simulink model "Ball_Estimation_10_12"  (Simulink 8.1)
settings: Solver=ode4  StartTime=0.0  StopTime=inf  FixedStep=sample_time  RelTol=1e-3
InitFcn:
  | sample_time=0.005;%0.004;%0.0025;%0.02;
  | sample_time_Vicon = 0.005;
  | DeltaT = 0.02;
  | g = 9.81;
  | H0 = g%0.3165;
  | Kl = 1;
  | 
  | Omega_r = 1.6;%for Horizontal reference
  | Zeta_r = 0.7; %for Horizontal reference
  | Omega = 1.8;%for Horizontal Control
  | Zeta = 0.5;    %for Horizontal Control
  | 
  | Omega_h_r = 2.2; %for vertical reference
  | Zeta_h_r = 0.8;  %for vertical reference
  | Omega_h = 2.3;    %for vertical control
  | Zeta_h = 0.8;         %for vertical control
  | PI=pi;
  | 
  | Mass = 1;
  | Acc_Max = 4;
  | Acc_Max_h = 4;
  | 
  | Max_RP = 60;
  | 
  | % for NN
  | n = 5;
  | r = 3;
  | n2 = 5;
  | NN_ST = 0.02;
  | 
  | GAMA_V = 6;
  | gama_V_e = 0.01;
  | 
  | GAMA_W = GAMA_V;
  | gama_W_e =0.01;
  | 
  | % deadzone
  | NN_Deadzone_Z = 0;
  | 
  | % inputs nomalizaton parameters
  | NN_Z_y_min = -3;
  | NN_Z_y_max = 0.5;
  | 
  | NN_Z_v_max = 8;
  | NN_Z_v_min = -NN_Z_v_max;
  | 
  | % alpha = 0.034;
  | alpha = 1;
  | % c_f = 0.0015;
  | c_f = 0.001;
  | c_y_tilt = 1*0.5;
undefined symbols (not defined in the file or in its folder): DiscIntNeverNeededParam
undefined symbols (not defined in the file): Q6_acc_max, Q6_acc_max_h, Q6_Omega_r, Q6_Omega_r_h, Q6_Zeta_r, Q6_Zeta_r_h
libraries: X330_Control x4, simulink x4
settings Model: Creator=ttcl3  LastModifiedBy=Vicon
settings SolverCC: MaxConsecutiveMinStep=auto
settings DebuggingCC: MultiTaskRateTransMsg=warning
settings SFSimCC: SimParseCustomCode=off

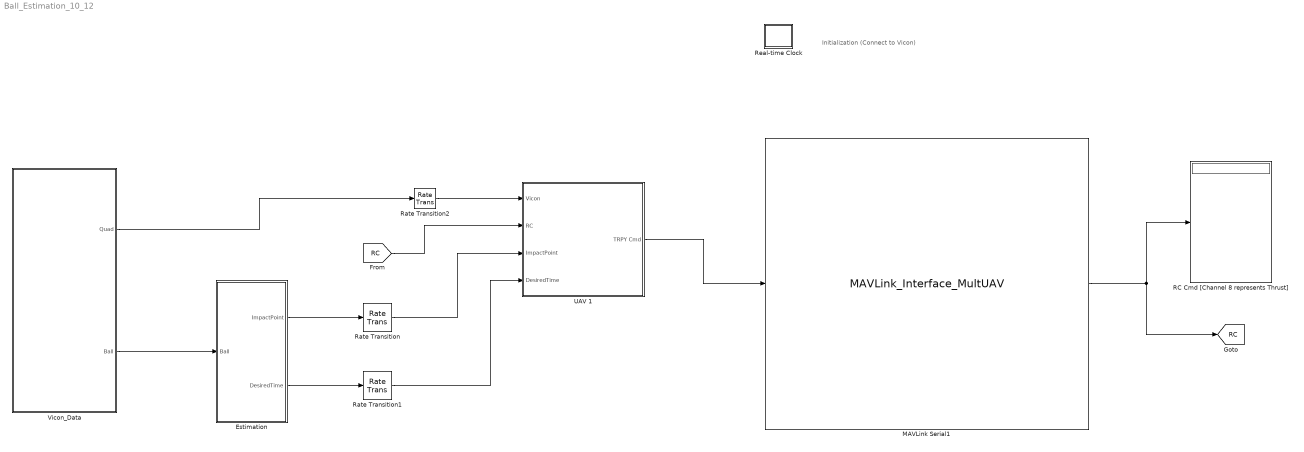
== system Ball_Estimation_10_12 ==
  note: Initialization
      | (Connect to Vicon)
  Estimation : Subsystem
  MAVLink Serial1 : S-Function  FunctionName=MAVLink_Interface_MultUAV  Parameters=COM_Port,Baud_Rate,MSG_INPUT,MSG_OUTPUT  EnableBusSupport=off  mask{COM_Port='COM5', Baud_Rate=57600, ATTITUDE_OUT=off, RC_SCALED=on, Quad_1=on, Quad_2=off, Quad_3=off, Quad_4=off, Quad_5=off, Quad_6=off, Quad_7=off, Quad_8=off, Quad_9=off, Quad_10=off, Quad_11=off, Quad_12=off, Quad_13=off, Quad_14=off, Quad_15=off, Quad_16=off, Quad_17=off, Quad_18=off, Quad_19=off, Quad_20=off, Quad_21=off, Quad_22=off, Quad_23=off, Quad_24=off, Quad_25=off, Quad_26=off, Quad_27=off, Quad_28=off, Quad_29=off, Quad_30=off}
      mask prompts: COM_Port "COM Port"; Baud_Rate "Baud Rate"; ATTITUDE_OUT "ATTITUDE"; RC_SCALED "RC CHANNELS SCALED"; Quad_1 "Quad No 1"; Quad_2 "Quad No 2"; Quad_3 "Quad No 3"; Quad_4 "Quad No 4"; Quad_5 "Quad No 5"; Quad_6 "Quad No 6"; Quad_7 "Quad No 7"; Quad_8 "Quad No 8"; Quad_9 "Quad No 9"; Quad_10 "Quad No 10"; Quad_11 "Quad No 11"; Quad_12 "Quad No 12"; Quad_13 "Quad No 13"; Quad_14 "Quad No 14"; Quad_15 "Quad No 15"; Quad_16 "Quad No 16"; Quad_17 "Quad No 17"; Quad_18 "Quad No 18"; Quad_19 "Quad No 19"; Quad_20 "Quad No 20"; Quad_21 "Quad No 21"; Quad_22 "Quad No 22"; Quad_23 "Quad No 23"; Quad_24 "Quad No 24"; Quad_25 "Quad No 25"; Quad_26 "Quad No 26"; Quad_27 "Quad No 27"; Quad_28 "Quad No 28"; Quad_29 "Quad No 29"; Quad_30 "Quad No 30"
      mask init:
      | MSG_ID_NUM_INPUT = [uint8(196) uint8(197) uint8(198) uint8(199) uint8(200) uint8(201) uint8(202) uint8(203) uint8(204) uint8(205)
      |                     uint8(206) uint8(207) uint8(208) uint8(209) uint8(210) uint8(211) uint8(212) uint8(213) uint8(214) uint8(215)
      |                     uint8(216) uint8(217) uint8(218) uint8(219) uint8(220) uint8(221) uint8(222) uint8(223) uint8(224) uint8(225)];
      | MSG_ID_NAME_INPUT = [Quad_1 Quad_2 Quad_3 Quad_4 Quad_5 Quad_6 Quad_7 Quad_8 Quad_9 Quad_10
      |                      Quad_11 Quad_12 Quad_13 Quad_14 Quad_15 Quad_16 Quad_17 Quad_18 Quad_19 Quad_20
      |                      Quad_21 Quad_22 Quad_23 Quad_24 Quad_25 Quad_26 Quad_27 Quad_28 Quad_29 Quad_30];
      | 
      | MSG_ID_NUM_OUTPUT = [uint8(34) uint8(30)];
      | MSG_ID_NAME_OUTPUT = [RC_SCALED ATTITUDE_OUT ];
      | 
      | idx_input = find(MSG_ID_NAME_INPUT);
      | MSG_INPUT = MSG_ID_NUM_INPUT(idx_input);
      | 
      | idx_output = find(MSG_ID_NAME_OUTPUT);
      | MSG_OUTPUT = MSG_ID_NUM_OUTPUT(idx_output);
      mask Display:
      | % Block image
      | image(imread('10-inch Quad Heat Map.png'));
      | 
      | %Label block
      | fprintf('MAVLink Serial\n%s\n%dbps', COM_Port,  Baud_Rate)
      | 
      | 
      | %Label input ports
      | 
      | in = 1;
      | if (Quad_1 == 1)
      |     port_label('input', in, 'Quad 1');
      |     in = in + 1;
      | end
      | if (Quad_2 == 1)
      |     port_label('input', in, 'Quad 2');
      |     in = in + 1;
      | end
      | 
      | if (Quad_3 == 1)
      |     port_label('input', in, 'Quad 3');
      |     in = in + 1;
      | end
      | 
      | if (Quad_4 == 1)
      |     port_label('input', in, 'Quad 4');
      |     in = in + 1;
      | end
      | 
      | if (Quad_5 == 1)
      |     port_label('input', in, 'Quad 5');
      |     in = in + 1;
      | end
      | 
      | if (Quad_6 == 1)
      |     port_label('input', in, 'Quad 6');
      |     in = in + 1;
      | end
      | 
      | if (Quad_7 == 1)
      |     port_label('input', in, 'Quad 7');
      |     in = in + 1;
      | end
      | 
      | if (Quad_8 == 1)
      |     port_label('input', in, 'Quad 8');
      |     in = in + 1;
      | end
      | 
      | if (Quad_9 == 1)
      |     port_label('input', in, 'Quad 9');
      |     in = in + 1;
      | end
      | 
      | if (Quad_10 == 1)
      |     port_label('input', in, 'Quad 10');
      |     in = in + 1;
      | end
      | 
      | if (Quad_11 == 1)
      |     port_label('input', in, 'Quad 11');
      |     in = in + 1;
      | end
      | 
      | if (Quad_12 == 1)
      |     port_label('input', in, 'Quad 12');
      |     in = in + 1;
      | end
      | 
      | if (Quad_13 == 1)
      |     port_label('input', in, 'Quad 13');
      |     in = in + 1;
      | end
      | 
      | if (Quad_14 == 1)
      |     port_label('input', in, 'Quad 14');
      |     in = in + 1;
      | end
      | 
      | if (Quad_15 == 1)
      |     port_label('input', in, 'Quad 15');
      |     in = in + 1;
      | end
      | 
      | if (Quad_16 == 1)
      |     port_label('input', in, 'Quad 16');
      |     in = in + 1;
      | end
      | 
      | if (Quad_17 == 1)
      |     port_label('input', in, 'Quad 17');
      |     in = in + 1;
      | end
      | 
      | if (Quad_18 == 1)
      |     port_label('input', in, 'Quad 18');
      |     in = in + 1;
      | end
      | 
      | 
      | if (Quad_19 == 1)
      |     port_label('input', in, 'Quad 19');
      |     in = in + 1;
      | end
      | 
      | if (Quad_20 == 1)
      |     port_label('input', in, 'Quad 20');
      |     in = in + 1;
      | end
      | 
      | if (Quad_21 == 1)
      |     port_label('input', in, 'Quad 21');
      |     in = in + 1;
      | end
      | 
      | if (Quad_22 == 1)
      |     port_label('input', in, 'Quad 22');
      |     in = in + 1;
      | end
      | 
      | if (Quad_23 == 1)
      |     port_label('input', in, 'Quad 23');
      |     in = in + 1;
      | end
      | 
      | if (Quad_24 == 1)
      |     port_label('input', in, 'Quad 24');
      |     in = in + 1;
      | end
      | 
      | if (Quad_25 == 1)
      |     port_label('input', in, 'Quad 25');
      |     in = in + 1;
      | end
      | 
      | if (Quad_26 == 1)
      |     port_label('input', in, 'Quad 26');
      |     in = in + 1;
      | end
      | 
      | if (Quad_27 == 1)
      |     port_label('input', in, 'Quad 27');
      |     in = in + 1;
      | end
      | 
      | if (Quad_28 == 1)
      |     port_label('input', in, 'Quad 28');
      |     in = in + 1;
      | end
      | 
      | if (Quad_29 == 1)
      |     port_label('input', in, 'Quad 29');
      |     in = in + 1;
      | end
      | 
      | if (Quad_30 == 1)
      |     port_label('input', in, 'Quad 30');
      |     in = in + 1;
      | end
      | %Label output ports
      | 
      | out = 1;
      | if (RC_SCALED == 1)
      |     port_label('output', out, 'RC CMD');
      |     out = out + 1;
      | end
      | 
      | if (ATTITUDE_OUT == 1)
      |     port_label('output', out, 'DEBUG');
      |     out = out + 1;
      | end
  RC Cmd [Channel 8 represents Thrust] : Display
  Rate Transition : RateTransition  OutPortSampleTime=0.02
  Rate Transition1 : RateTransition  OutPortSampleTime=0.02
  Rate Transition2 : RateTransition  OutPortSampleTime=0.02
  Real-time Clock : Subsystem  mask(Real-time Clock){sample_time=0.02, tolerance=1}
      mask prompts: sample_time "Synchronize with real-time every n seconds:"; tolerance "Real-time warning tolerance (seconds):"
      mask help: Real-time Synchronization Block
      mask Help: This block synchronizes simulation time with the PC real-time clock or UNIX system clock. The first dialog entry is the period at which the clock is checked to insure real-time synchronization. The second dialog entry is the number of seconds that the simulation time must be within real-time before a warning is printed.
      mask Display: plot(0,0,100,100,[40,60,60,54,54,64,69,76,82,77,81,83,83,81,78,74,70,64,57,49,41,35,32,30,30,31,34,40,47,47,40,40],[90,90,85,85,80,79,76,87,80,70,64,57,49,41,33,28,24,22,21,23,25,31,37,46,56,65,73,78,80,85,85,90],[69,53,53],[64,50,73])
  UAV 1 : Subsystem
  Vicon_Data : Subsystem
  tag scope: RC=global
  wires:
  Estimation/1(ImpactPoint) -> Rate Transition/1
  Estimation/2(DesiredTime) -> Rate Transition1/1
  [RC] -> UAV 1/2(RC)
  Rate Transition2/1 -> UAV 1/1(Vicon)
  MAVLink Serial1/1 -> [RC], RC Cmd [Channel 8 represents Thrust]/1
  UAV 1/1(TRPY Cmd) -> MAVLink Serial1/1
  Vicon_Data/2(Ball) -> Estimation/1(Ball)
  Vicon_Data/1(Quad) -> Rate Transition2/1
  Rate Transition/1 -> UAV 1/3(ImpactPoint)
  Rate Transition1/1 -> UAV 1/4(DesiredTime)

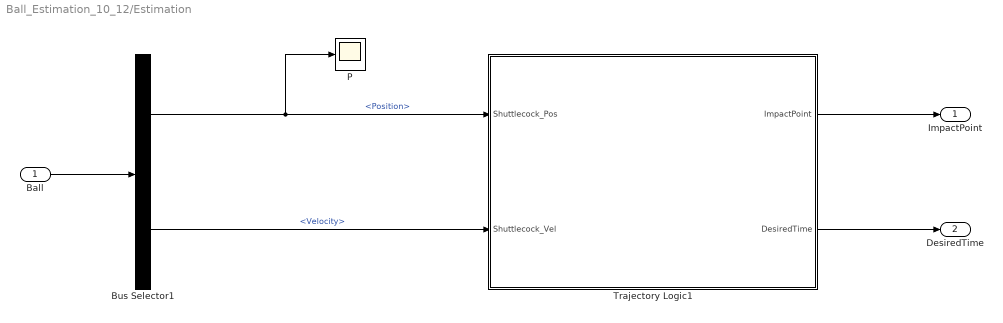
== system Ball_Estimation_10_12/Estimation ==
  Ball : Inport
  Bus Selector1 : BusSelector  OutputSignals=Position,Velocity
  P : Scope
      settings: MaxDataPoints=50000
  Trajectory Logic1 : Subsystem
  ImpactPoint : Outport
  DesiredTime : Outport  Port=2
  wires:
  Ball/1 -> Bus Selector1/1
  Bus Selector1/1 -> P/1, Trajectory Logic1/1(Shuttlecock_Pos)  "<Position>"
  Bus Selector1/2 -> Trajectory Logic1/2(Shuttlecock_Vel)  "<Velocity>"
  Trajectory Logic1/1("ImpactPoint ") -> ImpactPoint/1
  Trajectory Logic1/2(DesiredTime) -> DesiredTime/1

== system Ball_Estimation_10_12/Real-time Clock ==
  Real-time Clock : S-Function  FunctionName=rtclock  Parameters=sample_time, tolerance  EnableBusSupport=off

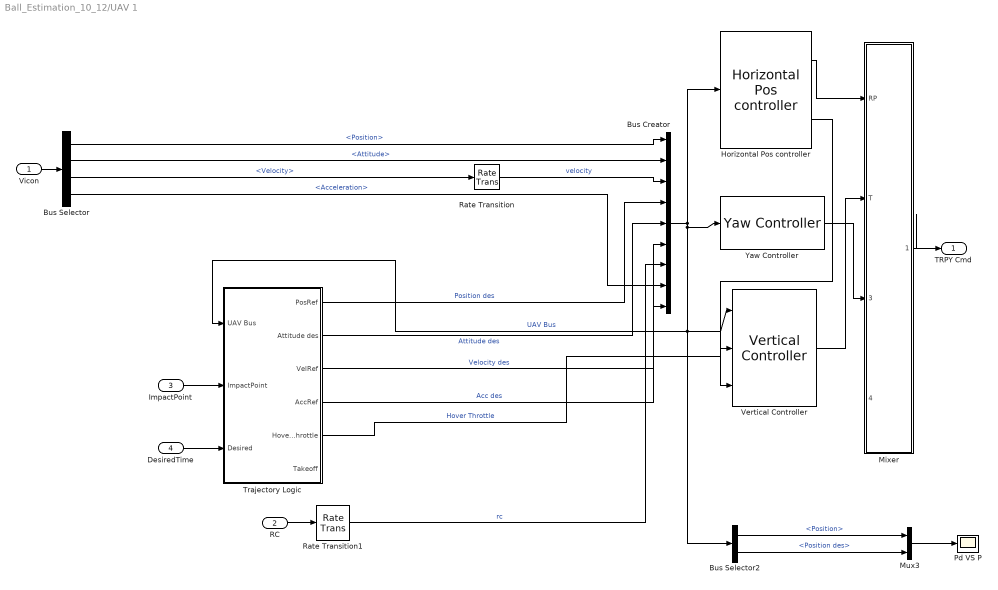
== system Ball_Estimation_10_12/UAV 1 ==
  Vicon : Inport
  RC : Inport  Port=2
  ImpactPoint : Inport  Port=3
  DesiredTime : Inport  Port=4
  Bus Creator : BusCreator  Inputs=9
  Bus Selector : BusSelector  OutputSignals=Position,Attitude,Velocity,Acceleration
  Bus Selector2 : BusSelector  OutputSignals=Position,Position des
  Horizontal Pos controller : X330_Control/Horizontal Pos controller  Max_RP=60  Omega=Q6_Omega  PID_i=1  Zeta=Q6_Zeta
  Mixer : Subsystem
  Mux3 : Mux  Inputs=2
  Pd VS P : Scope
      settings: TimeRange=10  YMin=-1  YMax=2.75
  Rate Transition : RateTransition  OutPortSampleTime=0.02
  Rate Transition1 : RateTransition  OutPortSampleTime=0.02
  Trajectory Logic : Subsystem
  Vertical Controller : X330_Control/Vertical Controller  Omega_h=Q6_Omega_h  Zeta_h=Q6_Zeta_h  PID_I_h=1  mass=Q6_mass
  Yaw Controller : X330_Control/Yaw Controller
  TRPY Cmd : Outport
  wires:
  Mux3/1 -> Pd VS P/1
  Bus Selector2/2 -> Mux3/2  "<Position des>"
  Bus Selector2/1 -> Mux3/1  "<Position>"
  Horizontal Pos controller/2 -> Vertical Controller/3
  RC/1 -> Rate Transition1/1
  Trajectory Logic/4(AccRef) -> Bus Creator/9  "Acc des"
  Mixer/1(XYZ RPY) -> TRPY Cmd/1
  Vicon/1 -> Bus Selector/1
  Bus Selector/3 -> Rate Transition/1  "<Velocity>"
  Bus Selector/2 -> Bus Creator/2  "<Attitude>"
  Bus Selector/1 -> Bus Creator/1  "<Position>"
  Trajectory Logic/5(HoverThrottle) -> Vertical Controller/2  "Hover Throttle"
  Trajectory Logic/3(VelRef) -> Bus Creator/6  "Velocity des"
  Trajectory Logic/2(Attitude des) -> Bus Creator/5  "Attitude des"
  Trajectory Logic/1(PosRef) -> Bus Creator/4  "Position des"
  Bus Selector/4 -> Bus Creator/8  "<Acceleration>"
  Vertical Controller/1 -> Mixer/2(T)
  Yaw Controller/1 -> Mixer/3(Yaw rate)
  Bus Creator/1 -> Yaw Controller/1, Bus Selector2/1, Vertical Controller/1, Trajectory Logic/1(UAV Bus), Horizontal Pos controller/1  "UAV Bus"
  Rate Transition1/1 -> Bus Creator/7  "rc"
  Rate Transition/1 -> Bus Creator/3  "velocity"
  Horizontal Pos controller/1 -> Mixer/1(RP)
  ImpactPoint/1 -> Trajectory Logic/2(ImpactPoint)
  DesiredTime/1 -> Trajectory Logic/3(Desired)

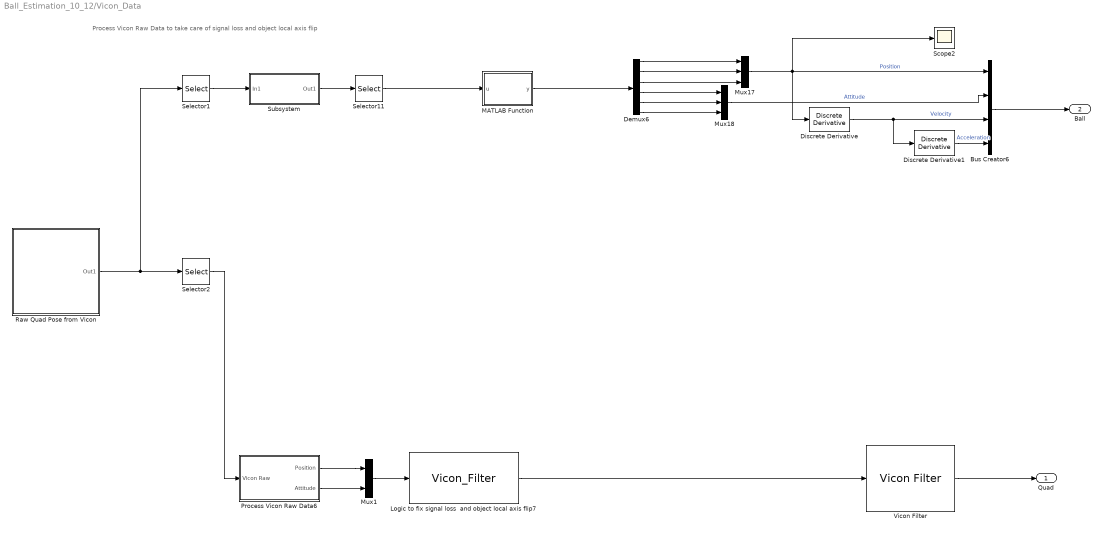
== system Ball_Estimation_10_12/Vicon_Data ==
  note: Process Vicon Raw Data to take care of signal loss and object local axis flip
  Bus Creator6 : BusCreator
  Demux6 : Demux  Outputs=6
  Discrete Derivative : simulink/Discrete/Discrete Derivative  gainval=1.0  ICPrevScaledInput=0.0  InputProcessing=Inherited  OutMin=[]  OutMax=[]  OutDataType=fixdt(1, 16)  OutScaling=2^-10  DoSatur=off
  Discrete Derivative1 : simulink/Discrete/Discrete Derivative  gainval=1.0  ICPrevScaledInput=0.0  InputProcessing=Inherited  OutMin=[]  OutMax=[]  OutDataType=fixdt(1, 16)  OutScaling=2^-10  DoSatur=off
  Logic to fix signal loss  and object local axis flip7 : M-S-Function  FunctionName=Vicon_Filter
  MATLAB Function : MATLAB Function  TreatAsAtomicUnit=on
  Mux1 : Mux  Inputs=2
  Mux17 : Mux  Inputs=3
  Mux18 : Mux  Inputs=3
  Process Vicon Raw Data6 : Subsystem
  Raw Quad Pose from Vicon : Subsystem
  Scope2 : Scope
      settings: YMin=-3  YMax=4.5
  Selector1 : Selector  InputPortWidth=12  IndexOptions=Index vector (dialog)  Indices=[7 8 9]  OutputSizes=1
  Selector11 : Selector  InputPortWidth=6  IndexOptions=Index vector (dialog)  Indices=[1 2 3 ]  OutputSizes=1
  Selector2 : Selector  InputPortWidth=12  IndexOptions=Index vector (dialog)  Indices=[1 2 3 4 5 6]  OutputSizes=1
  Subsystem : Subsystem
  Vicon Filter : X330_Control/Vicon Filter
  Quad : Outport
  Ball : Outport  Port=2
  wires:
  Demux6/6 -> Mux18/3
  Mux17/1 -> Scope2/1, Bus Creator6/1, Discrete Derivative/1  "Position"
  Raw Quad Pose from Vicon/1(Out1) -> Selector2/1, Selector1/1
  Selector1/1 -> Subsystem/1(In1)
  MATLAB Function/1(y) -> Demux6/1
  Subsystem/1(Out1) -> Selector11/1
  Selector11/1 -> MATLAB Function/1(u)
  Demux6/5 -> Mux18/2
  Demux6/4 -> Mux18/1
  Mux18/1 -> Bus Creator6/2  "Attitude"
  Demux6/1 -> Mux17/1
  Demux6/2 -> Mux17/2
  Demux6/3 -> Mux17/3
  Discrete Derivative/1 -> Discrete Derivative1/1, Bus Creator6/3  "Velocity"
  Discrete Derivative1/1 -> Bus Creator6/4  "Acceleration"
  Selector2/1 -> Process Vicon Raw Data6/1(Vicon Raw)
  Logic to fix signal loss  and object local axis flip7/1 -> Vicon Filter/1
  Process Vicon Raw Data6/1(Position) -> Mux1/1
  Process Vicon Raw Data6/2(Attitude) -> Mux1/2
  Mux1/1 -> Logic to fix signal loss  and object local axis flip7/1
  Vicon Filter/1 -> Quad/1
  Bus Creator6/1 -> Ball/1

== system Ball_Estimation_10_12/Estimation/Trajectory Logic1 ==
  Shuttlecock_Pos : Inport
  Shuttlecock_Vel : Inport  Port=2
  ImpactPoint1 : Scope
      settings: YMin=-4  YMax=4  SaveName=ScopeData2  MaxDataPoints=50000
  UAV SF : Stateflow chart  TreatAsAtomicUnit=on
  "ImpactPoint " : Outport
  DesiredTime : Outport  Port=2
  wires:
  Shuttlecock_Pos/1 -> UAV SF/1(Sc_Pos)
  Shuttlecock_Vel/1 -> UAV SF/2(Sc_Vel)
  UAV SF/1(ImpactPoint) -> "ImpactPoint "/1, ImpactPoint1/1
  UAV SF/2(DesiredTime) -> DesiredTime/1

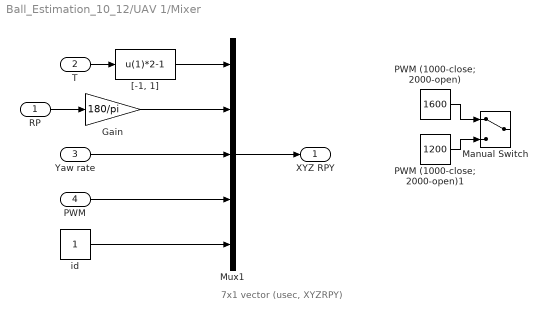
== system Ball_Estimation_10_12/UAV 1/Mixer ==
  note: 7x1 vector (usec, XYZRPY)
  RP : Inport
  T : Inport  Port=2
  Yaw rate : Inport  Port=3
  PWM : Inport  Port=4
  Gain : Gain  Gain=180/pi
  Manual Switch : ManualSwitch
  Mux1 : Mux  Inputs=5
  PWM (1000-close; 2000-open) : Constant  Value=1600  SampleTime=0.02
  PWM (1000-close; 2000-open)1 : Constant  Value=1200  SampleTime=0.02
  "[-1, 1]" : Fcn  Expr=u(1)*2-1
  id : Constant  SampleTime=0.02
  XYZ RPY : Outport
  wires:
  "[-1, 1]"/1 -> Mux1/1
  Gain/1 -> Mux1/2
  PWM/1 -> Mux1/4
  PWM (1000-close; 2000-open)1/1 -> Manual Switch/2
  PWM (1000-close; 2000-open)/1 -> Manual Switch/1
  id/1 -> Mux1/5
  Yaw rate/1 -> Mux1/3
  RP/1 -> Gain/1
  T/1 -> "[-1, 1]"/1
  Mux1/1 -> XYZ RPY/1

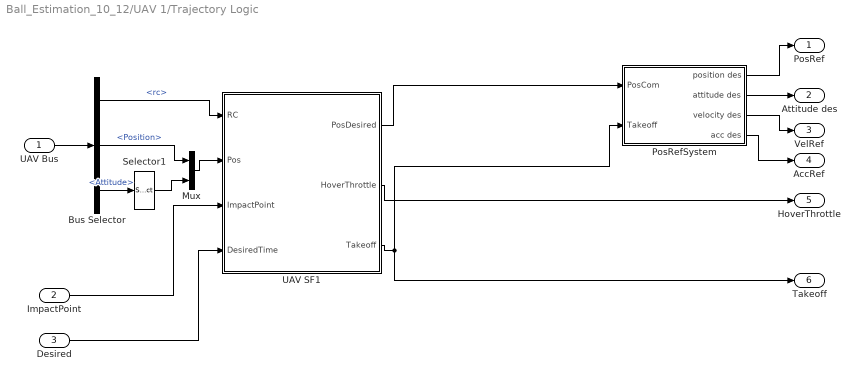
== system Ball_Estimation_10_12/UAV 1/Trajectory Logic ==
  UAV Bus : Inport
  ImpactPoint : Inport  Port=2
  Desired : Inport  Port=3
  Bus Selector : BusSelector  OutputSignals=rc,Position,Attitude
  Mux : Mux  Inputs=2
  PosRefSystem : Subsystem  AncestorBlock=X330_Control/PosRefSystem  mask{Omega_r=Q6_Omega_r, Zeta_r=Q6_Zeta_r, Acc_Max=Q6_acc_max, Omega_h_r=Q6_Omega_r_h, Zeta_h_r=Q6_Zeta_r_h, Acc_h_Max=Q6_acc_max_h}
      mask prompts: Omega_r "Omega_r (P Gain= Omega_r^2)"; Zeta_r "Zeta_r (D = 2*Omega_r*Zeta_r)"
  Selector1 : Selector  InputPortWidth=3  IndexOptions=Index vector (dialog)  Indices=[3]  OutputSizes=1
  UAV SF1 : Stateflow chart  TreatAsAtomicUnit=on
  PosRef : Outport
  Attitude des : Outport  Port=2
  VelRef : Outport  Port=3
  AccRef : Outport  Port=4
  HoverThrottle : Outport  Port=5
  Takeoff : Outport  Port=6
  wires:
  PosRefSystem/2(attitude des) -> Attitude des/1
  PosRefSystem/4(acc des) -> AccRef/1
  PosRefSystem/3(velocity des) -> VelRef/1
  PosRefSystem/1(position des) -> PosRef/1
  Mux/1 -> UAV SF1/2(Pos)
  Selector1/1 -> Mux/2
  Bus Selector/3 -> Selector1/1  "<Attitude>"
  Bus Selector/2 -> Mux/1  "<Position>"
  UAV Bus/1 -> Bus Selector/1
  ImpactPoint/1 -> UAV SF1/3(ImpactPoint)
  UAV SF1/2(HoverThrottle) -> HoverThrottle/1
  Bus Selector/1 -> UAV SF1/1(RC)  "<rc>"
  UAV SF1/1(PosDesired) -> PosRefSystem/1(PosCom)
  UAV SF1/3(Takeoff) -> Takeoff/1, PosRefSystem/2(Takeoff)
  Desired/1 -> UAV SF1/4(DesiredTime)

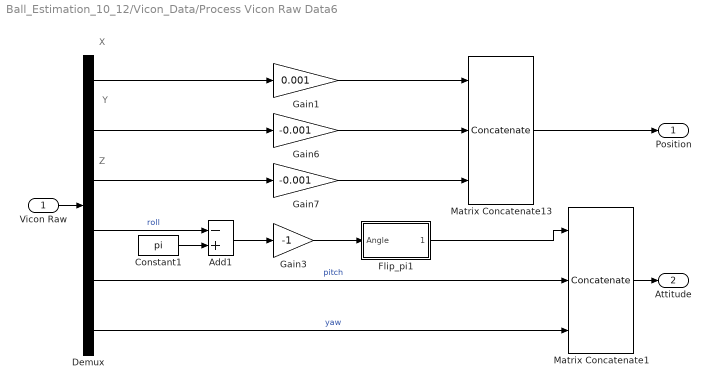
== system Ball_Estimation_10_12/Vicon_Data/Process Vicon Raw Data6 ==
  note: X
  note: Y
  note: Z
  Vicon Raw : Inport
  Add1 : Sum  Inputs=-+
  Constant1 : Constant  Value=pi  OutDataTypeStr=double
  Demux : Demux  Outputs=6
  Flip_pi1 : Subsystem  mask(Flip -pi to pi){}
      mask help: Flips the inputs into the range -pi to pi
      mask Help: Flips the inputs into the range -pi to pi
      mask Display: disp('Flip_pi')
  Gain1 : Gain  Gain=0.001
  Gain3 : Gain  Gain=-1
  Gain6 : Gain  Gain=-0.001
  Gain7 : Gain  Gain=-0.001
  Matrix Concatenate1 : Concatenate  NumInputs=3  Mode=Multidimensional array
  Matrix Concatenate13 : Concatenate  NumInputs=3  Mode=Multidimensional array
  Position : Outport
  Attitude : Outport  Port=2
  wires:
  Constant1/1 -> Add1/2
  Demux/6 -> Matrix Concatenate1/3  "yaw"
  Gain1/1 -> Matrix Concatenate13/1
  Demux/1 -> Gain1/1
  Demux/2 -> Gain6/1
  Demux/3 -> Gain7/1
  Demux/4 -> Add1/1  "roll"
  Gain6/1 -> Matrix Concatenate13/2
  Gain7/1 -> Matrix Concatenate13/3
  Add1/1 -> Gain3/1
  Gain3/1 -> Flip_pi1/1(Angle)
  Demux/5 -> Matrix Concatenate1/2  "pitch"
  Flip_pi1/1(Angle_Flip) -> Matrix Concatenate1/1
  Matrix Concatenate13/1 -> Position/1
  Vicon Raw/1 -> Demux/1
  Matrix Concatenate1/1 -> Attitude/1

== system Ball_Estimation_10_12/Vicon_Data/Raw Quad Pose from Vicon ==
  Constant : Constant
  Interpreted MATLAB Function : MATLABFcn  MATLABFcn=GetViconPose_MAV1  OutputDimensions=12  SampleTime=0.005
  Out1 : Outport
  wires:
  Constant/1 -> Interpreted MATLAB Function/1
  Interpreted MATLAB Function/1 -> Out1/1

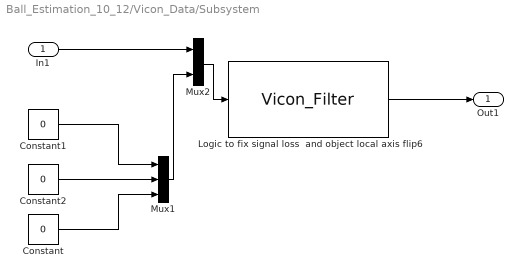
== system Ball_Estimation_10_12/Vicon_Data/Subsystem ==
  In1 : Inport
  Constant : Constant  Value=0
  Constant1 : Constant  Value=0
  Constant2 : Constant  Value=0
  Logic to fix signal loss  and object local axis flip6 : M-S-Function  FunctionName=Vicon_Filter
  Mux1 : Mux  Inputs=3
  Mux2 : Mux  Inputs=2
  Out1 : Outport
  wires:
  Constant1/1 -> Mux1/1
  Constant2/1 -> Mux1/2
  Mux1/1 -> Mux2/2
  Mux2/1 -> Logic to fix signal loss  and object local axis flip6/1
  Constant/1 -> Mux1/3
  In1/1 -> Mux2/1
  Logic to fix signal loss  and object local axis flip6/1 -> Out1/1

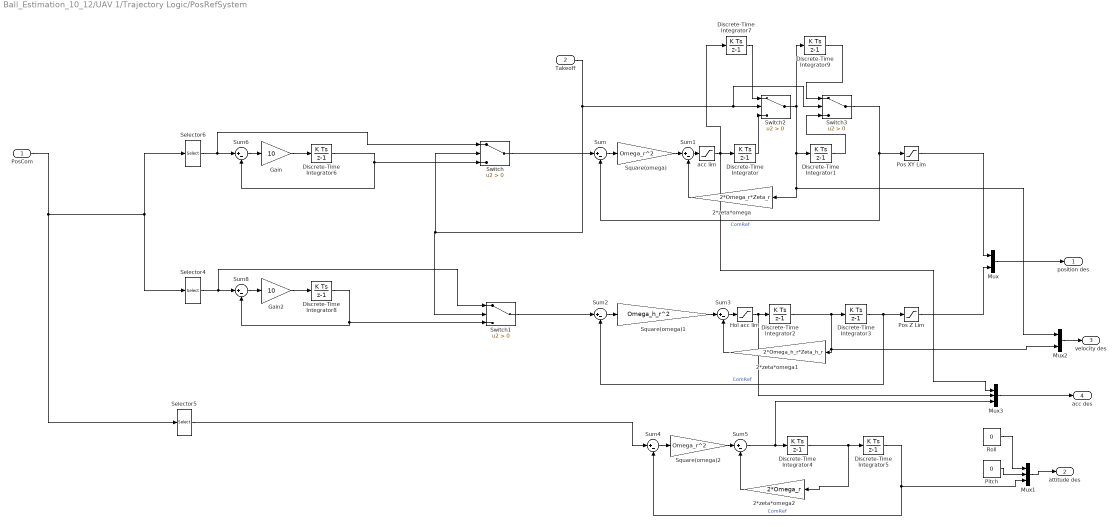
== system Ball_Estimation_10_12/UAV 1/Trajectory Logic/PosRefSystem ==
  PosCom : Inport
  Takeoff : Inport  Port=2
  2*zeta*omega : Gain  Gain=2*Omega_r*Zeta_r
  2*zeta*omega1 : Gain  Gain=2*Omega_h_r*Zeta_h_r
  2*zeta*omega2 : Gain  Gain=2*Omega_r
  Discrete-Time Integrator{,1..2,7,9} (5 alike) : DiscreteIntegrator  gainval=1  SampleTime=-1  ICPrevOutput=DiscIntNeverNeededParam  ICPrevScaledInput=DiscIntNeverNeededParam
  Discrete-Time Integrator{3..6,8} (5 alike) : DiscreteIntegrator  SampleTime=-1  ICPrevOutput=DiscIntNeverNeededParam  ICPrevScaledInput=DiscIntNeverNeededParam
  Gain : Gain  Gain=10
  Gain2 : Gain  Gain=10
  Hol acc lim : Saturate  UpperLimit=Acc_h_Max  LowerLimit=-Acc_h_Max
  Mux : Mux  Inputs=2
  Mux1 : Mux  Inputs=3
  Mux2 : Mux  Inputs=2
  Mux3 : Mux  Inputs=3
  Pitch : Constant  Value=0  SampleTime=0.02
  Pos XY Lim : Saturate  UpperLimit=3  LowerLimit=-3
  Pos Z Lim : Saturate  LowerLimit=-3
  Roll : Constant  Value=0  SampleTime=0.02
  Selector4 : Selector  InputPortWidth=4  IndexOptions=Index vector (dialog)  Indices=[3]  OutputSizes=1
  Selector5 : Selector  InputPortWidth=4  IndexOptions=Index vector (dialog)  Indices=[4]  OutputSizes=1
  Selector6 : Selector  InputPortWidth=4  IndexOptions=Index vector (dialog)  Indices=[1 2]  OutputSizes=1
  Square(omega) : Gain  Gain=Omega_r^2
  Square(omega)1 : Gain  Gain=Omega_h_r^2
  Square(omega)2 : Gain  Gain=Omega_r^2
  Sum{,1..6,8} (8 alike) : Sum  Inputs=|+-
  Switch{,1..3} (4 alike) : Switch  Criteria=u2 > Threshold
  acc lim : Saturate  UpperLimit=Acc_Max  LowerLimit=-Acc_Max
  position des : Outport
  attitude des : Outport  Port=2
  velocity des : Outport  Port=3
  acc des : Outport  Port=4
  wires:
  Pos Z Lim/1 -> Mux/2
  Pos XY Lim/1 -> Mux/1
  Sum8/1 -> Gain2/1
  Gain2/1 -> Discrete-Time Integrator8/1
  Discrete-Time Integrator8/1 -> Switch1/3, Sum8/2
  Sum6/1 -> Gain/1
  Gain/1 -> Discrete-Time Integrator6/1
  Discrete-Time Integrator6/1 -> Switch/3, Sum6/2
  Mux3/1 -> acc des/1
  Mux2/1 -> velocity des/1
  Mux1/1 -> attitude des/1
  Pitch/1 -> Mux1/2
  Roll/1 -> Mux1/1
  Mux/1 -> position des/1
  Switch3/1 -> Pos XY Lim/1, Sum/2  "ComRef"
  Selector5/1 -> Sum4/1
  2*zeta*omega2/1 -> Sum5/2
  Sum5/1 -> Mux3/3, Discrete-Time Integrator4/1
  Discrete-Time Integrator4/1 -> 2*zeta*omega2/1, Discrete-Time Integrator5/1
  Square(omega)2/1 -> Sum5/1
  Sum4/1 -> Square(omega)2/1
  Discrete-Time Integrator5/1 -> Mux1/3, Sum4/2  "ComRef"
  Hol acc lim/1 -> Mux3/2, Discrete-Time Integrator2/1
  2*zeta*omega1/1 -> Sum3/2
  Sum3/1 -> Hol acc lim/1
  Discrete-Time Integrator2/1 -> Mux2/2, 2*zeta*omega1/1, Discrete-Time Integrator3/1
  Square(omega)1/1 -> Sum3/1
  Sum2/1 -> Square(omega)1/1
  Discrete-Time Integrator3/1 -> Pos Z Lim/1, Sum2/2  "ComRef"
  acc lim/1 -> Discrete-Time Integrator7/1, Mux3/1, Discrete-Time Integrator/1
  2*zeta*omega/1 -> Sum1/2
  Sum1/1 -> acc lim/1
  Switch2/1 -> Mux2/1, 2*zeta*omega/1, Discrete-Time Integrator1/1, Discrete-Time Integrator9/1
  Square(omega)/1 -> Sum1/1
  Sum/1 -> Square(omega)/1
  Takeoff/1 -> Switch3/2, Switch2/2, Switch1/2, Switch/2
  PosCom/1 -> Selector4/1, Selector6/1, Selector5/1
  Switch/1 -> Sum/1
  Switch1/1 -> Sum2/1
  Selector6/1 -> Switch/1, Sum6/1
  Selector4/1 -> Switch1/1, Sum8/1
  Discrete-Time Integrator/1 -> Switch2/3
  Discrete-Time Integrator7/1 -> Switch2/1
  Discrete-Time Integrator9/1 -> Switch3/1
  Discrete-Time Integrator1/1 -> Switch3/3

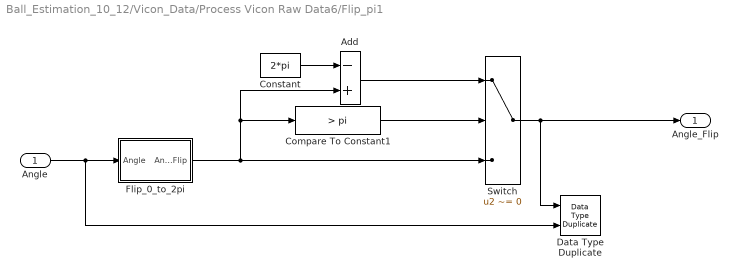
== system Ball_Estimation_10_12/Vicon_Data/Process Vicon Raw Data6/Flip_pi1 ==
  Angle : Inport
  Add : Sum  Inputs=-+
  Compare To Constant1 : simulink/Logic and Bit Operations/Compare To Constant  relop=>  const=pi  OutDataTypeStr=uint8  ZeroCross=off
  Constant : Constant  Value=2*pi
  Data Type Duplicate : DataTypeDuplicate
  Flip_0_to_2pi : Subsystem  mask(Flip zero to 2pi){}
      mask help: Flips the inputs into the range zero to +2pi
      mask Help: Flips the inputs into the range zero to +2pi
      mask Display: disp('Flip_0_2pi')
  Switch : Switch  Criteria=u2 ~= 0
  Angle_Flip : Outport
  wires:
  Switch/1 -> Data Type Duplicate/1, Angle_Flip/1
  Add/1 -> Switch/1
  Constant/1 -> Add/1
  Compare To Constant1/1 -> Switch/2
  Flip_0_to_2pi/1(Angle_Flip) -> Add/2, Compare To Constant1/1, Switch/3
  Angle/1 -> Data Type Duplicate/2, Flip_0_to_2pi/1(Angle)

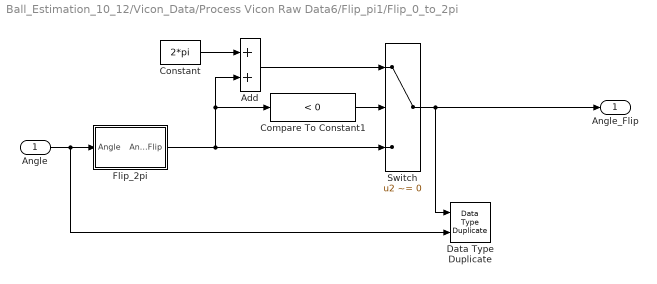
== system Ball_Estimation_10_12/Vicon_Data/Process Vicon Raw Data6/Flip_pi1/Flip_0_to_2pi ==
  Angle : Inport
  Add : Sum
  Compare To Constant1 : simulink/Logic and Bit Operations/Compare To Constant  relop=<  const=0  OutDataTypeStr=uint8  ZeroCross=off
  Constant : Constant  Value=2*pi
  Data Type Duplicate : DataTypeDuplicate
  Flip_2pi : Subsystem  mask(Flip -2pi to 2pi){}
      mask help: Flips the inputs into the range -2pi to +2pi
      mask Help: Flips the inputs into the range -2pi to +2pi
      mask Display: disp('Flip_2pi')
  Switch : Switch  Criteria=u2 ~= 0
  Angle_Flip : Outport
  wires:
  Switch/1 -> Data Type Duplicate/1, Angle_Flip/1
  Angle/1 -> Data Type Duplicate/2, Flip_2pi/1(Angle)
  Add/1 -> Switch/1
  Constant/1 -> Add/1
  Compare To Constant1/1 -> Switch/2
  Flip_2pi/1(Angle_Flip) -> Switch/3, Add/2, Compare To Constant1/1

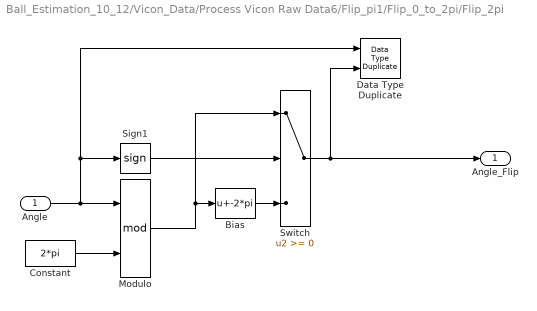
== system Ball_Estimation_10_12/Vicon_Data/Process Vicon Raw Data6/Flip_pi1/Flip_0_to_2pi/Flip_2pi ==
  Angle : Inport
  Bias : Bias  Bias=-2*pi
  Constant : Constant  Value=2*pi
  Data Type Duplicate : DataTypeDuplicate
  Modulo : Math  Operator=mod  SaturateOnIntegerOverflow=on
  Sign1 : Signum
  Switch : Switch
  Angle_Flip : Outport
  wires:
  Switch/1 -> Data Type Duplicate/2, Angle_Flip/1
  Bias/1 -> Switch/3
  Sign1/1 -> Switch/2
  Modulo/1 -> Switch/1, Bias/1
  Constant/1 -> Modulo/2
  Angle/1 -> Data Type Duplicate/1, Sign1/1, Modulo/1

== matlab function Vicon_Data/MATLAB Function ==
  data: u input double; y output double
function y = fcn(u)
%#codegen
y = zeros(6,1);
y(1) = u(1)/1000;
y(2) = -u(2)/1000;
y(3) = -u(3)/1000;
y(4) = 0;
y(5) = 0;
y(6) = 0;
end

== stateflow chart Estimation/Trajectory Logic1/UAV SF ==
  state Airborne
    state Standby
    state Calculation
      en:
      [Pe,T]=TrajEst(x,y,z,zd,Peo[0],Peo[1],To);
      x[0] = x[1];x[1] = x[2];x[2] = x[3];x[3] = x[4];
      y[0] = y[1];y[1] = y[2];y[2] = y[3];y[3] = y[4];
      z[0] = z[1];z[1] = z[2];z[2] = z[3];z[3] = z[4];
    state Getdata
      en:
      x[i] = Sc_Pos[0];
      y[i] = Sc_Pos[1];
      z[i] = Sc_Pos[2];
    state Output1
      en:
      ImpactPoint = Pe;
      DesiredTime = T;
    state daq
      en:
      i=i+1;
    (default) -> Standby : {i=-1;Peo=0;To=0;}
    Standby -> (junction 17) : [(abs(Sc_Pos[0]) <= 4.5)&(abs(Sc_Pos[1])<=4.5)&(abs(Sc_Pos[2])<=4)]
    (junction 17) -> daq [order 1] : [(Sc_Vel[2] < -1)&(Sc_Vel[2] > -6)&(Sc_Pos[2] <-0.5)]
    (junction 17) -> Standby [order 2]
    Getdata -> daq
    daq -> Getdata [order 1] : [i==0]
    (junction 18) -> Getdata [order 1] : [(x[i-1]~=Sc_Pos[0])||(y[i-1]~=Sc_Pos[1])||(z[i-1]~=Sc_Pos[2])]
    Output1 -> daq : {i=i-2;}
    daq -> (junction 18) [order 3] : [(i>0)&(i<5)]
    (junction 18) -> daq [order 2] : {i=i-1;}
    daq -> Calculation [order 2] : [i==5]
    Calculation -> Output1 : {Peo=Pe;To=T;}
  data: xi function_input double size=5; yi function_input double size=5; zi function_input double size=5; Pe function_output double size=3; T function_output double size=1; zd function_input double size=1; t0 constant double size=5 =[0 0.02 0.04 0.06 0.08]; xo function_input double; yo function_input double; To function_input double; ImpactPoint output double size=3; DesiredTime output double size=1; Sc_Pos input double size=3; Sc_Vel input double size=3; DeltaT parameter double size=1; T local double size=1; zd local double size=1 =-0.5; Pe local double size=3; i local double; x local double size=5 =[0 0 0 0 0]; y local double size=5 =[0 0 0 0 0]; z local double size=5 =[0 0 0 0 0]; Peo local double size=3; To local double size=1
  function [Pe,T]=TrajEst(xi,yi,zi,zd,xo,yo,To):
    | function [Pe,T]=TrajEst(xi,yi,zi,zd,xo,yo,To)
    | 
    | p=polyfit(t0,zi,2)';
    | a=p(1);
    | b=p(2);
    | c=p(3);
    | 
    | 
    | xe=0;
    | ye=0;
    | T=0;
    | if((To>0)&&(To<1.2))
    |     xe = xo;
    |     ye = yo;
    |     T = To;
    | end;
    | if(a > 3)
    |     if(b^2 - 4*a*(c-zd) >= 0)
    |         T=(-b+sqrt(b^2 - 4*a*(c-zd)))/(2*a);
    |         xe=polyval(polyfit(t0,xi,1),T);
    |         ye=polyval(polyfit(t0,yi,1),T);
    |     end;
    | 
    |     if((To>0)&&(To<1.2))
    |         if((T>1.2)||(abs(xe)>4)||(abs(ye)>4))
    |             T = To;
    |             xe = xo;
    |             ye = yo;
    |         else
    |             T = 0.7*T + 0.3*(To-0.005);
    |             xe = 0.7*xo + 0.3*xe;
    |             ye = 0.7*yo + 0.3*ye;
    |         end
    |     else
    |        if((T>1.2)||(abs(xe)>4)||(abs(ye)>4)) 
    |            xe=0;
    |            ye=0;
    |            T=0;
    |        end;
    |     end;
    | end
    | 
    | Pe=[xe ye zd]';

== stateflow chart UAV 1/Trajectory Logic/UAV SF1 ==
  state Landing
    state Decsending
      en:PosDesired = Pos;
      du:PosDesired[2] = (0 - PosDesired[2])*1*DeltaT + PosDesired[2] ;
    state CutThrottle
      du:HoverThrottle = (0.01 - HoverThrottle)*2*DeltaT + HoverThrottle ;
    (default) -> Decsending
    Decsending -> CutThrottle : [Pos[2] > -0.15]
  state Airborne1
    state TakeOff
      du:HoverThrottle = (H0 - HoverThrottle)*2*DeltaT + HoverThrottle ;
    state Hover
      en: PosDesired[2] = -1;takeoff=0;
    state Trajectory
      state Line1
        en: PosDesired[0] = 2; PosDesired[1] = 0; PosDesired[2] = -1;takeoff=1;
      state Line2
        en: PosDesired[0] = -2; PosDesired[1] = 0; PosDesired[2] = -1;takeoff=1;
      (default) -> Line1 : {line_count = -1;}
      Line1 -> Line2 : after (6, sec)
      Line2 -> Line1 : after (6, sec)
    (default) -> TakeOff [order 2] : {PosDesired = Pos;  PosDesired[2] = -1;takeoff=0;}
    TakeOff -> Hover : after(5,sec)
        | {PosDesired = Pos;}
    Hover -> (junction 68) : [(ImpactPoint[0] ~= 0)&(ImpactPoint[1]~= 0)]
    (default) -> Hover [order 1] : [RC[5] < 0]
        | {PosDesired = Pos;}
  Landing -> Airborne1 : [RC[6] > 0.5]
  Airborne1 -> Landing : [RC[6] < -0.5]
  (default) -> Landing : {HoverThrottle=0.01;}
  data: PosDesired output double size=4; HoverThrottle output double size=1; RC input double size=8; Pos input double size=4; ImpactPoint input double size=3; DeltaT parameter double size=1; H0 parameter double size=1; Kl parameter double size=1; zmax constant double size=1 =-2.5; Takeoff output double size=1; DesiredTime input double size=1; xmax constant double size=1 =3; xmin constant double size=1 =-3; ymax constant double size=1 =3; ymin constant double size=1 =-3; data local double
